simulink model "windup_discrete_spring16"  (R2015b)
settings: Solver=VariableStepAuto  StartTime=0.0  StopTime=20  RelTol=1e-3
values from neighbouring files (symbols this model uses):
  h = 0.05    [BLDC_partial2_fall18.m]    (also in abs_spring18.m = 0.2; active_suspension_ss.m = 0.00416985950901; active_suspension_ss_R.m = 0.00416985950901; active_suspension_ss_spring18.m = 0.004)
  K = 10    [abs_spring18.m]    (also in double_integrator_deadbeat.m = [2;1]; harddisk_discrete_design.m = 20; harddisk_discrete_design_2dof_example.m = 20; hw_tank_simulink_pid_tuning.m = 0.575539568345)
  N = 400    [MR2007_final_fall18.m]    (also in covfcn.m = length(x); hw_tank_simulink_pid_tuning.m = 10; tanker_yaw_unstable.m = 20)
  Td = 0:h:0.5    [active_suspension_ss.m]    (also in active_suspension_ss_R.m; active_suspension_ss_spring18.m; final_dummy.m = 1; hw_tank_simulink_pid_tuning.m = 1.42361065574)
  Ti = 2*L    (= 5.69444262295)    [hw_tank_simulink_pid_tuning.m]
undefined symbols (not defined in the file or in its folder): A1, A2, B1, B2, uHigh, uLow
settings Model: Creator=kjartan  LastModifiedBy=kjartan

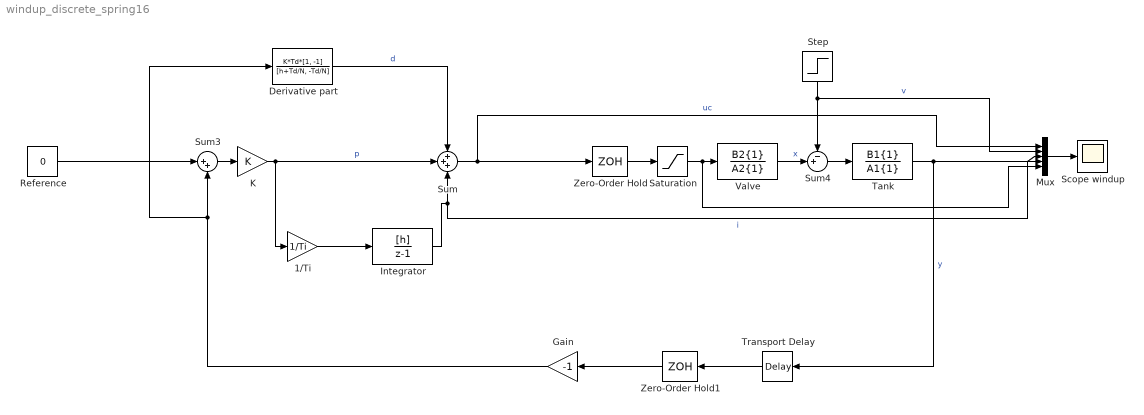
== system windup_discrete_spring16 ==
  1/Ti : Gain  Gain=1/Ti
  Derivative part : DiscreteFilter  Numerator=K*Td*[1, -1]  Denominator=[h+Td/N, -Td/N]  SampleTime=h
  Gain : Gain  Gain=-1
  Integrator : DiscreteTransferFcn  Numerator=[h]  Denominator=[1 -1]  SampleTime=h
  K : Gain  Gain=K
  Mux : Mux  Inputs=5
  Reference : Constant  Value=0
  Saturation : Saturate  UpperLimit=uHigh  LowerLimit=uLow
  Scope windup : Scope
  Step : Step  Time=5  SampleTime=0
  Sum : Sum  Inputs=+++
  Sum3 : Sum  Inputs=|++
  Sum4 : Sum  Inputs=-+|
  Tank : TransferFcn  Numerator=B1{1}  Denominator=A1{1}
  Transport Delay : TransportDelay  DelayTime=0.1
  Valve : TransferFcn  Numerator=B2{1}  Denominator=A2{1}
  Zero-Order Hold : ZeroOrderHold  SampleTime=h
  Zero-Order Hold1 : ZeroOrderHold  SampleTime=h
  wires:
  Sum/1 -> Zero-Order Hold/1, Mux/1  "uc"
  Derivative part/1 -> Sum/1  "d"
  K/1 -> 1/Ti/1, Sum/2  "p"
  Integrator/1 -> Sum/3, Mux/4  "i"
  Reference/1 -> Sum3/1
  Sum3/1 -> K/1
  Mux/1 -> Scope windup/1
  Gain/1 -> Derivative part/1, Sum3/2
  Zero-Order Hold1/1 -> Gain/1
  Saturation/1 -> Mux/5, Valve/1
  Step/1 -> Mux/2, Sum4/1  "v"
  Sum4/1 -> Tank/1
  Tank/1 -> Transport Delay/1, Mux/3  "y"
  Transport Delay/1 -> Zero-Order Hold1/1
  Zero-Order Hold/1 -> Saturation/1
  Valve/1 -> Sum4/2  "x"
  1/Ti/1 -> Integrator/1
